simulink model "PIEstimator"  (Simulink 10.0)
settings: Solver=ode3  StartTime=0.0  StopTime=Tsim  FixedStep=deltat  RelTol=1e-3  EnableMultiTasking=on
values from neighbouring files (symbols this model uses):
  a = 1    [estimator_params_pi.m]    (also in params.m = 0.00588235294118)
  alpha2 = 3    [estimator_params_pi.m]
  delay = 0.01    [estimator_params_pi.m]    (also in estimator_params_pid.m)
  deltat = 0.001    [estimator_params_pi.m]    (also in estimator_params_pid.m)
  K1 = 10    [estimator_params_pi.m]    (also in estimator_params_pid.m = 5)
  K2 = 30    [estimator_params_pi.m]    (also in estimator_params_pid.m = 2.121)
  Tsim = 20    [estimator_params_pi.m]    (also in estimator_params_pid.m)
  umax = 41.9*0.85    (= 35.615)    [estimator_params_pi.m]    (also in estimator_params_pid.m = 4.59)
  umin = -9    [estimator_params_pi.m]    (also in estimator_params_pid.m = -24.735)
settings Model: Creator=e50128  LastModifiedBy=adityaaaap
settings DataIOCC: LimitDataPoints=on  SignalLoggingSaveFormat=ModelDataLogs
settings OptimizationCC: ExpressionDepthLimit=2147483647
settings DebuggingCC: SolverPrmCheckMsg=warning  FcnCallInpInsideContextMsg=warning  StateNameClashWarn=warning
settings GRTTargetCC: GeneratePreprocessorConditionals=Disable all
settings ConfigComp: CovExternalEMLEnable=off

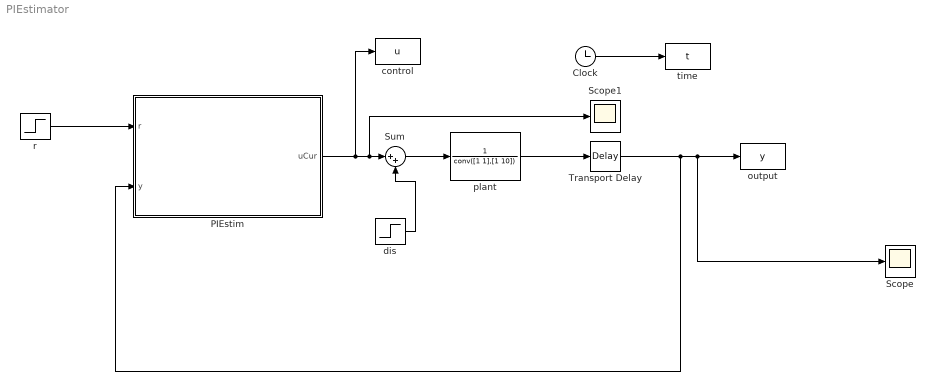
== system PIEstimator ==
  Clock : Clock
  PIEstim : MATLAB Function  TreatAsAtomicUnit=on
  Scope : Scope
  Scope1 : Scope
  Sum : Sum  Inputs=|++
  Transport Delay : TransportDelay  DelayTime=delay
  control : ToWorkspace  VariableName=u
      settings: MaxDataPoints=100000
  dis : Step  Time=Tsim/2  After=20  SampleTime=0
  output : ToWorkspace  VariableName=y
      settings: MaxDataPoints=100000
  plant : TransferFcn  Denominator=conv([1 1],[1 10])
  r : Step  Time=0  SampleTime=0
  time : ToWorkspace  VariableName=t
      settings: MaxDataPoints=100000
  wires:
  r/1 -> PIEstim/1(r)
  Clock/1 -> time/1
  plant/1 -> Transport Delay/1
  Transport Delay/1 -> Scope/1, output/1, PIEstim/2(y)
  PIEstim/1(uCur) -> Scope1/1, Sum/1, control/1
  dis/1 -> Sum/2
  Sum/1 -> plant/1

== matlab function PIEstim ==
  settings: updateMethod=DISCRETE  sampleTime=deltat
  data: uCur output double; r input double; y input double; K1 parameter double; K2 parameter double; alpha2 parameter double; a parameter double; deltat parameter double; umin parameter double; umax parameter double
function uCur = PIEstim(r,y,K1,K2,alpha2,a,deltat,umin,umax)
persistent zhat
if isempty(zhat)
    zhat=0;
end
%estimator based MATLAB function with anti-windup
dhat=zhat+K2*(y-r);
uCur= -K1*(y-r)-dhat; 
if (uCur>umax) uCur=umax;end
if (uCur<umin) uCur=umin;end
%zhat=zhat-alpha2*zhat*deltat-deltat*(y-r)*K2*(alpha2-a)-deltat*alpha2*udelay(1,ndmax);
zhat=zhat-alpha2*zhat*deltat-deltat*(y-r)*K2*(alpha2-a)-deltat*alpha2*uCur;
